simulink model "Day_09_Method1"  (R2024a)
settings: Solver=FixedStepAuto  StartTime=0.0  StopTime=10  FixedStep=0.01  RelTol=1e-3
values from neighbouring files (symbols this model uses):
  D0 = 2700    [Day_09.m]
  D1 = 2700    [Day_09.m]
  disturbance = 0    [Day_09.m]
  L0 = 0.01    [Day_09.m]
  L1 = 0.14    [Day_09.m]
  lim_theta = 2*pi    (= 6.28318530718)    [Day_09.m]
  lim_u = 1    [Day_09.m]
  lim_x = 1    [Day_09.m]
  M0 = L0*W0*T0*D0    (= 0.0027)    [Day_09.m]
  M1 = L1*W1*T1*D1    (= 0.0378)    [Day_09.m]
  M_c = 5    [Day_09.m]
  N_p = 50    [Day_09.m]
  num_state = 2    [Day_09.m]
  Q_Bar = kron(eye(N_p), Q)    [Day_09.m]
  R_Bar = kron(eye(M_c), R)    [Day_09.m]
  T0 = 0.01    [Day_09.m]
  T1 = 0.01    [Day_09.m]
  T_s = 0.01    [Day_09.m]
  Trajectory = zeros(num_state, 20000)    [Day_09.m]
  W0 = 0.01    [Day_09.m]
  W1 = 0.01    [Day_09.m]
undefined symbols (not defined in the file or in its folder): X, Y, Z
libraries: sm_lib x14, nesl_utility x7, simulink x1
settings Model: Creator=mingeun  LastModifiedBy=MinGeunPark
settings SolverCC: ZeroCrossAlgorithm=Adaptive
settings DataIOCC: ReturnWorkspaceOutputs=off
settings OptimizationCC: BlockReduction=off  DefaultParameterBehavior=Inlined  BufferReuse=off
settings DebuggingCC: IgnoredZcDiagnostic=none

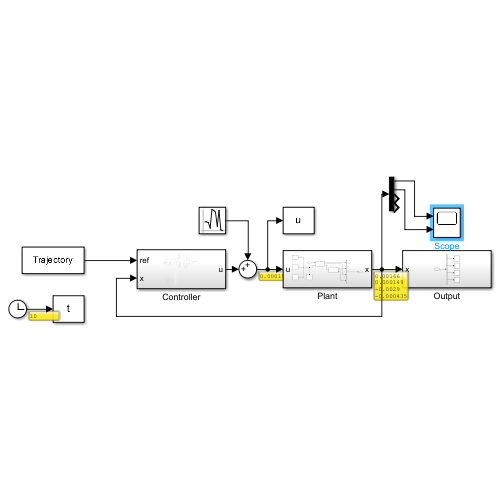
[thumbnail: Simulink's stored preview of the top-level diagram]
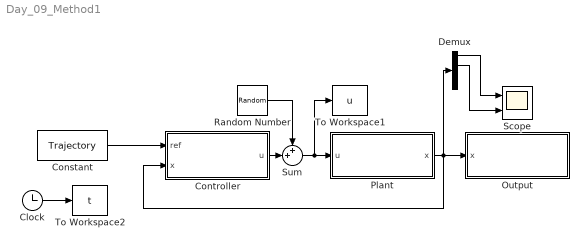
== system Day_09_Method1 ==
  Clock : Clock
  Constant : Constant  Value=Trajectory
  Controller : Subsystem
  Demux : Demux
  Output : Subsystem
  Plant : Subsystem
  Random Number : RandomNumber  Variance=0  SampleTime=T_s
  Scope : Scope  NumInputPorts=2
  Sum : Sum  Inputs=++|
  To Workspace1 : ToWorkspace  VariableName=u  SampleTime=-1
  To Workspace2 : ToWorkspace  VariableName=t  SampleTime=-1
  wires:
  Clock/1 -> To Workspace2/1
  Constant/1 -> Controller/1(ref)
  Plant/1(x) -> Demux/1, Controller/2(x), Output/1(x)
  Controller/1(u) -> Sum/2
  Sum/1 -> To Workspace1/1, Plant/1(u)
  Demux/1 -> Scope/1
  Demux/2 -> Scope/2
  Random Number/1 -> Sum/1

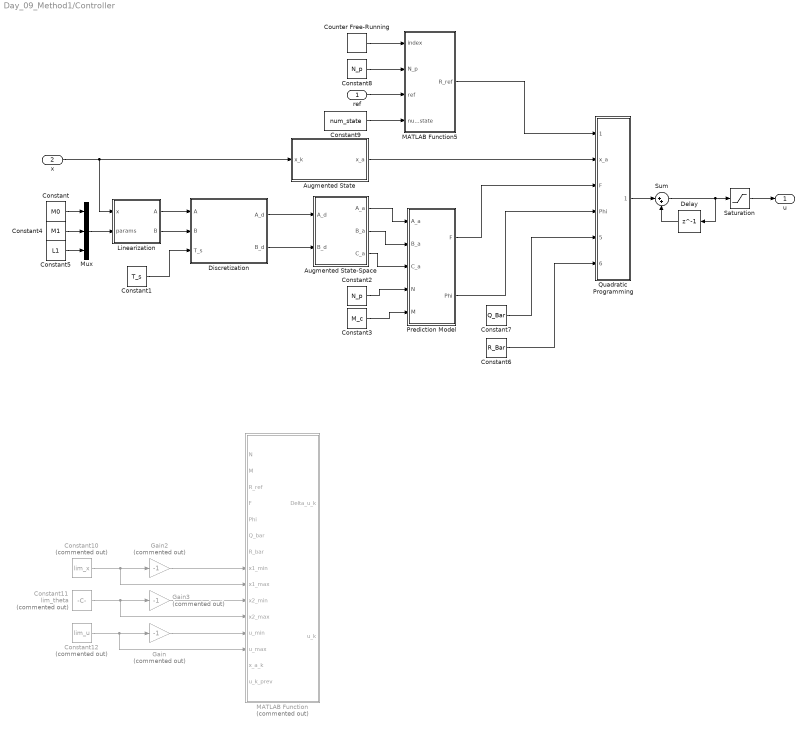
== system Day_09_Method1/Controller ==
  ref : Inport
  x : Inport  Port=2
  Augmented State : Subsystem
  Augmented State-Space : MATLAB Function  TreatAsAtomicUnit=on
  Constant : Constant  Value=M0
  Constant1 : Constant  Value=T_s
  Constant10 : Constant  Commented=on  Value=lim_x
  Constant11 : Constant  Commented=on  Value=lim_theta
  Constant12 : Constant  Commented=on  Value=lim_u
  Constant2 : Constant  Value=N_p
  Constant3 : Constant  Value=M_c
  Constant4 : Constant  Value=M1
  Constant5 : Constant  Value=L1
  Constant6 : Constant  Value=R_Bar
  Constant7 : Constant  Value=Q_Bar
  Constant8 : Constant  Value=N_p
  Constant9 : Constant  Value=num_state
  Counter Free-Running : simulink/Sources/Counter Free-Running  NumBits=32  tsamp=T_s
  Delay : Delay  DelayLength=1
  Discretization : Subsystem
  Gain : Gain  Commented=on  Gain=-1
  Gain2 : Gain  Commented=on  Gain=-1
  Gain3 : Gain  Commented=on  Gain=-1
  Linearization : MATLAB Function  TreatAsAtomicUnit=on
  MATLAB Function : MATLAB Function  Commented=on  TreatAsAtomicUnit=on
  MATLAB Function5 : MATLAB Function  TreatAsAtomicUnit=on
  Mux : Mux  Inputs=3
  Prediction Model : MATLAB Function  TreatAsAtomicUnit=on
  Quadratic Programming : Subsystem
  Saturation : Saturate  UpperLimit=lim_u  LowerLimit=-lim_u
  Sum : Sum  Inputs=|++
  u : Outport
  wires:
  Constant4/1 -> Mux/2
  Constant/1 -> Mux/1
  Sum/1 -> Saturation/1, Delay/1
  ref/1 -> MATLAB Function5/3(ref)
  Constant1/1 -> Discretization/3(T_s)
  Constant9/1 -> MATLAB Function5/4(num_state)
  Linearization/1(A) -> Discretization/1(A)
  Linearization/2(B) -> Discretization/2(B)
  Delay/1 -> Sum/2
  Prediction Model/2(Phi) -> Quadratic Programming/4(Phi)
  Augmented State/1(x_a) -> Quadratic Programming/2(x_a)
  Constant7/1 -> Quadratic Programming/5(Q_Bar)
  Counter Free-Running/1 -> MATLAB Function5/1(index)
  Constant8/1 -> MATLAB Function5/2(N_p)
  x/1 -> Linearization/1(x), Augmented State/1(x_k)
  MATLAB Function5/1(R_ref) -> Quadratic Programming/1(R_ref)
  Augmented State-Space/3(C_a) -> Prediction Model/3(C_a)
  Constant6/1 -> Quadratic Programming/6(R_Bar)
  Constant2/1 -> Prediction Model/4(N)
  Augmented State-Space/2(B_a) -> Prediction Model/2(B_a)
  Prediction Model/1(F) -> Quadratic Programming/3(F)
  Discretization/1(A_d) -> Augmented State-Space/1(A_d)
  Mux/1 -> Linearization/2(params)
  Augmented State-Space/1(A_a) -> Prediction Model/1(A_a)
  Discretization/2(B_d) -> Augmented State-Space/2(B_d)
  Constant3/1 -> Prediction Model/5(M)
  Constant5/1 -> Mux/3
  Constant12/1 -> MATLAB Function/13(u_max), Gain/1
  Constant10/1 -> MATLAB Function/9(x1_max), Gain2/1
  Gain2/1 -> MATLAB Function/8(x1_min)
  Gain3/1 -> MATLAB Function/10(x2_min)
  Constant11/1 -> MATLAB Function/11(x2_max), Gain3/1
  Gain/1 -> MATLAB Function/12(u_min)
  Saturation/1 -> u/1
  Quadratic Programming/1(Delta_u) -> Sum/1

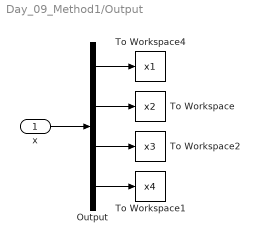
== system Day_09_Method1/Output ==
  x : Inport
  Output : Demux
  To Workspace : ToWorkspace  VariableName=x2  SampleTime=-1
  To Workspace1 : ToWorkspace  VariableName=x4  SampleTime=-1
  To Workspace2 : ToWorkspace  VariableName=x3  SampleTime=-1
  To Workspace4 : ToWorkspace  VariableName=x1  SampleTime=-1
  wires:
  Output/3 -> To Workspace2/1
  Output/4 -> To Workspace1/1
  Output/2 -> To Workspace/1
  Output/1 -> To Workspace4/1
  x/1 -> Output/1

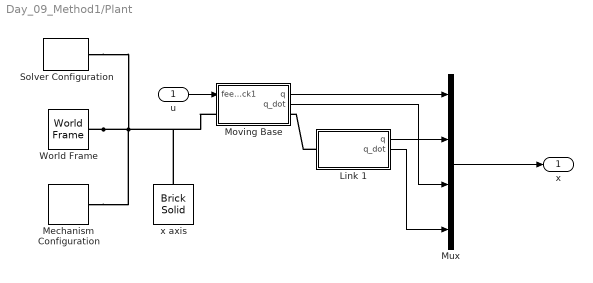
== system Day_09_Method1/Plant ==
  u : Inport
  Link 1 : Subsystem  mask{L=L1*100, W=W1*100, H=T1*100, rho=D1, rgb=[0.25 0.40 0.70], angle=0, F=disturbance}
      mask prompts: L "Length (cm)"; W "Width (cm)"; H "Thickness (cm)"; rho "Density (kg/m^3)"; rgb "Color [R G B]"; angle "Initial Angle (degree)"; F "Disturbance [N]"
  Mechanism Configuration : sm_lib/Utilities/Mechanism Configuration  UniformGravity=Constant  GravityVector=[0 0 -9.81]  GravityVectorUnits=m/s^2  LinearizationDelta=0.001  JointModeTransitionNonlinearIterations=2
  Moving Base : Subsystem  mask{L=L0*100, W=W0*100, H=T0*100, rho=D0, RGB=[0.8 0.45 0.0], x_init=0}
      mask prompts: L "Length (cm)"; W "Width (cm)"; H "Thickness (cm)"; rho "Density (kg/m^3)"; RGB "Color [R G B]"; x_init "x_init (cm)"
  Mux : Mux
  Solver Configuration : nesl_utility/Solver Configuration  PhysicalDomain=network_engine_domain  SubClassName=solver  LeftPortType=input  RightPortType=generic  Tones=[]  Harmonics=[]  SimulateNoise=off  Profile=off  UseLocalSampling=off  EnableSwitchedLinearOptims=on  FrequencyDomain=off  UseCCode=off  RelTol=0.001  AbsTol=0.001  MinStep=1e-09  ToWorkspace=off  RevertToSquareIcSolve=off  NumHomotopyIterations=100  PhasorMode=off  PhasorModeNumHarmonics=1  ConsistencySolver=NEWTON_XTOL_AFTER_FTOL  IndexReductionMethod=DerivativeReplacement  DoDC=off  ResidualTolerance=1e-09  ConsistencyTolSource=GLOBAL  ConsistencyAbsTol=0.001  ConsistencyRelTol=0.001  ConsistencyTolFactor=0.001  UseLocalSolver=off  LocalSolverChoice=NE_BACKWARD_EULER_ADVANCER  ResolveIndetEquations=on  FunctionEvalNumThread=1  LocalSolverSampleTime=0.001  DoFixedCost=off  MaxNonlinIter=3  MaxModeIter=2  ComputeImpulses=off  ImpulseIterations=2  LinearAlgebra=auto  LinearAlgebraNumThread=0  EquationFormulation=NE_TIME_EF  DelaysMemoryBudget=1024  AutomaticFiltering=on  FilteringTimeConstant=0.001  PartitionStorageMethod=AS_NEEDED  PartitionMemoryBudget=1024  PartitionMethod=ROBUST  MultibodyUseLocalSolver=off  MultibodyLocalSolverChoice=ODE1  MultibodyLocalSolverSampleTime=0.001
  World Frame : sm_lib/Frames and Transforms/World Frame
  x axis : sm_lib/Body Elements/Brick Solid  BrickDimensions=[1000 1 1]  BrickDimensionsUnits=mm  ExportEntireGeometry=off  InertiaType=CalculateFromGeometry  BasedOnType=Density  Density=1000  DensityUnits=kg/m^3  Mass=1  MassUnits=kg  CenterOfMass=[0 0 0]  CenterOfMassUnits=m  MomentsOfInertia=[1 1 1]  MomentsOfInertiaUnits=kg*m^2  ProductsOfInertia=[0 0 0]  ProductsOfInertiaUnits=kg*m^2  GraphicType=FromGeometry  MarkerShape=Sphere  MarkerSize=10  GraphicVisPropType=SimpleVisualProperties  GraphicDiffuseColor=[0.0 0.0 0.0]  GraphicOpacity=1  GraphicSpecularColor=[0.5 0.5 0.5 1.0]  GraphicAmbientColor=[0.15 0.15 0.15 1.0]  GraphicEmissiveColor=[0.0 0.0 0.0 1.0]  GraphicShininess=75  DoExposeReferenceFrame=on  SerializedFrames=<Frames/>
  x : Outport
  wires:
  Moving Base/1(q) -> Mux/1
  Link 1/1(q) -> Mux/2
  u/1 -> Moving Base/1(feedback1)
  Link 1/2(q_dot) -> Mux/4
  Moving Base/2(q_dot) -> Mux/3
  Mux/1 -> x/1
  connections:
  World Frame/RConn1 -- Solver Configuration/RConn1 -- Moving Base/LConn1 -- x axis/RConn1 -- Mechanism Configuration/RConn1
  Link 1/LConn1 -- Moving Base/RConn1

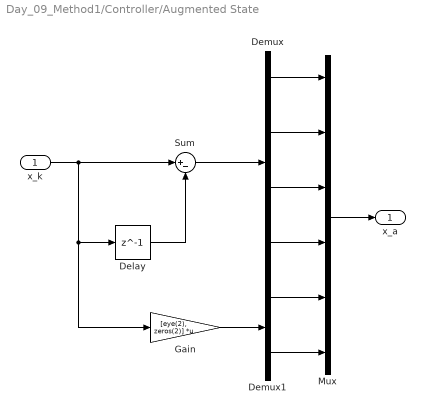
== system Day_09_Method1/Controller/Augmented State ==
  x_k : Inport
  Delay : Delay  DelayLength=1
  Demux : Demux
  Demux1 : Demux  Outputs=2
  Gain : Gain  Gain=[eye(2), zeros(2)]  Multiplication=Matrix(K*u) (u vector)
  Mux : Mux  Inputs=6
  Sum : Sum  Inputs=|+-
  x_a : Outport
  wires:
  x_k/1 -> Sum/1, Gain/1, Delay/1
  Sum/1 -> Demux/1
  Demux/1 -> Mux/1
  Demux/2 -> Mux/2
  Demux/3 -> Mux/3
  Demux/4 -> Mux/4
  Demux1/1 -> Mux/5
  Demux1/2 -> Mux/6
  Mux/1 -> x_a/1
  Delay/1 -> Sum/2
  Gain/1 -> Demux1/1

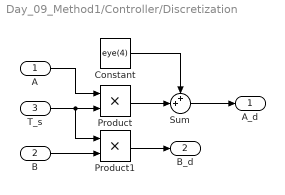
== system Day_09_Method1/Controller/Discretization ==
  A : Inport
  B : Inport  Port=2
  T_s : Inport  Port=3
  Constant : Constant  Value=eye(4)
  Product : Product
  Product1 : Product
  Sum : Sum  Inputs=++|
  A_d : Outport
  B_d : Outport  Port=2
  wires:
  Sum/1 -> A_d/1
  Product1/1 -> B_d/1
  Constant/1 -> Sum/1
  B/1 -> Product1/2
  T_s/1 -> Product1/1, Product/2
  Product/1 -> Sum/2
  A/1 -> Product/1

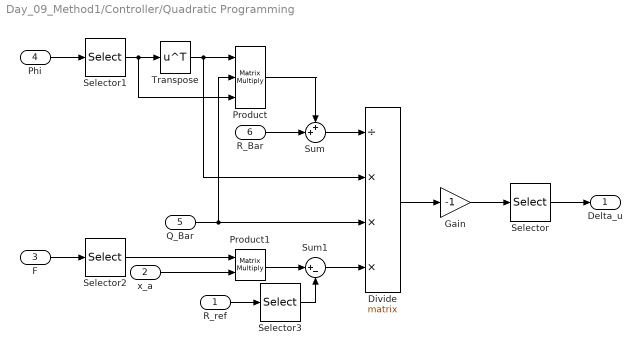
== system Day_09_Method1/Controller/Quadratic Programming ==
  R_ref : Inport
  x_a : Inport  Port=2
  F : Inport  Port=3
  Phi : Inport  Port=4
  Q_Bar : Inport  Port=5
  R_Bar : Inport  Port=6
  Divide : Product  Inputs=/***  Multiplication=Matrix(*)
  Gain : Gain  Gain=-1
  Product : Product  Inputs=3  Multiplication=Matrix(*)
  Product1 : Product  Multiplication=Matrix(*)
  Selector : Selector  InputPortWidth=M_c  IndexOptions=Index vector (dialog)  Indices=1  OutputSizes=1
  Selector1 : Selector  NumberOfDimensions=2  InputPortWidth=3  IndexOptions=Index vector (dialog),Index vector (dialog)  Indices=[1:N_p*num_state],[1:M_c]  OutputSizes=1,1
  Selector2 : Selector  NumberOfDimensions=2  InputPortWidth=3  IndexOptions=Index vector (dialog),Index vector (dialog)  Indices=[1:N_p*num_state],[1:4 + num_state]  OutputSizes=1,1
  Selector3 : Selector  NumberOfDimensions=2  InputPortWidth=N_p*2  IndexOptions=Index vector (dialog),Index vector (dialog)  Indices=[1:N_p*num_state],1  OutputSizes=1,1
  Sum : Sum  Inputs=++|
  Sum1 : Sum  Inputs=|+-
  Transpose : Math  Operator=transpose
  Delta_u : Outport
  wires:
  Selector/1 -> Delta_u/1
  Gain/1 -> Selector/1
  Divide/1 -> Gain/1
  Sum1/1 -> Divide/4
  Product1/1 -> Sum1/1
  Sum/1 -> Divide/1
  R_Bar/1 -> Sum/2
  F/1 -> Selector2/1
  Product/1 -> Sum/1
  Q_Bar/1 -> Product/2, Divide/3
  Transpose/1 -> Divide/2, Product/1
  Phi/1 -> Selector1/1
  Selector1/1 -> Product/3, Transpose/1
  Selector2/1 -> Product1/1
  R_ref/1 -> Selector3/1
  Selector3/1 -> Sum1/2
  x_a/1 -> Product1/2

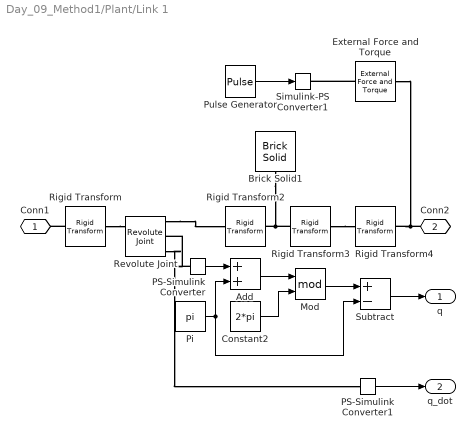
== system Day_09_Method1/Plant/Link 1 ==
  Add : Sum
  Brick Solid1 : sm_lib/Body Elements/Brick Solid  BrickDimensions=[L W H]  BrickDimensionsUnits=cm  ExportEntireGeometry=off  InertiaType=CalculateFromGeometry  BasedOnType=Density  Density=rho  DensityUnits=kg/m^3  Mass=1  MassUnits=kg  CenterOfMass=[0 0 0]  CenterOfMassUnits=m  MomentsOfInertia=[1 1 1]  MomentsOfInertiaUnits=kg*m^2  ProductsOfInertia=[0 0 0]  ProductsOfInertiaUnits=kg*m^2  GraphicType=FromGeometry  MarkerShape=Sphere  MarkerSize=10  GraphicVisPropType=SimpleVisualProperties  GraphicDiffuseColor=rgb  GraphicOpacity=1  GraphicSpecularColor=[0.5 0.5 0.5 1.0]  GraphicAmbientColor=[0.15 0.15 0.15 1.0]  GraphicEmissiveColor=[0.0 0.0 0.0 1.0]  GraphicShininess=75  DoExposeReferenceFrame=on  SerializedFrames=<Frames/>
  Constant2 : Constant  Value=2*pi
  External Force and Torque : sm_lib/Forces and Torques/External Force and Torque  EnableForceX=on  EnableForceY=off  EnableForceZ=off  EnableForce=off  ForceResolutionFrame=World  EnableTorqueX=off  EnableTorqueY=off  EnableTorqueZ=off  EnableTorque=off  TorqueResolutionFrame=World
  Mod : Math  Operator=mod  OutputSignalType=real
  PS-Simulink Converter : nesl_utility/PS-Simulink Converter  PhysicalDomain=network_engine_domain  SubClassName=ps_output  LeftPortType=input  RightPortType=output  PseudoPeriodic=off  Frequencies=[]  VectorFormat=inherit  Unit=inherit  AffineConversion=off
  PS-Simulink Converter1 : nesl_utility/PS-Simulink Converter  PhysicalDomain=network_engine_domain  SubClassName=ps_output  LeftPortType=input  RightPortType=output  PseudoPeriodic=off  Frequencies=[]  VectorFormat=inherit  Unit=inherit  AffineConversion=off
  Pi : Constant  Value=pi  OutDataTypeStr=Inherit: Inherit via back propagation
  Pulse Generator : DiscretePulseGenerator  PulseType=Time based  Amplitude=F  Period=1000000  PulseWidth=1/1000000  PhaseDelay=0.25
  Revolute Joint : sm_lib/Joints/Revolute Joint  JointMode=Normal  CompositeWrenchDir=FollowerOnBase  CompositeWrenchFrame=BaseFrame  SenseConstraintForce=off  SenseConstraintTorque=off  SenseTotalForce=off  SenseTotalTorque=off  PositionTargetSpecify=on  PositionTargetPriority=High  PositionTargetValue=angle  PositionTargetValueUnits=deg  VelocityTargetSpecify=off  VelocityTargetPriority=High  VelocityTargetValue=0  VelocityTargetValueUnits=deg/s  EquilibriumPosition=0  EquilibriumPositionUnits=deg  SpringStiffness=0  SpringStiffnessUnits=N*m/deg  DampingCoefficient=0  DampingCoefficientUnits=N*m/(deg/s)  LowerLimitSpecify=off  LowerLimitBound=-90  LowerLimitBoundUnits=deg  LowerLimitStiffness=1e4  LowerLimitStiffnessUnits=N*m/deg  LowerLimitDamping=10  LowerLimitDampingUnits=N*m/(deg/s)  LowerLimitTransitionRegionWidth=0.1  LowerLimitTransitionRegionWidthUnits=deg  UpperLimitSpecify=off  UpperLimitBound=90  UpperLimitBoundUnits=deg  UpperLimitStiffness=1e4  UpperLimitStiffnessUnits=N*m/deg  UpperLimitDamping=10  UpperLimitDampingUnits=N*m/(deg/s)  UpperLimitTransitionRegionWidth=0.1  UpperLimitTransitionRegionWidthUnits=deg  TorqueActuationMode=InputTorque  MotionActuationMode=ComputedMotion  SensePosition=on  SenseVelocity=on  SenseAcceleration=off  SenseTorqueForce=off  SenseLowerLimitTorqueForce=off  SenseUpperLimitTorqueForce=off
  Rigid Transform : sm_lib/Frames and Transforms/Rigid Transform  RotationMethod=RotationMatrix  FollAlignAxisA=+X  BaseAlignAxisA=+Y  FollAlignAxisB=+Y  BaseAlignAxisB=+Z  RotationStandardAxis=+X  RotationAngle=90  RotationAngleUnits=deg  RotationArbitraryAxis=[0 0 1]  RotationSequenceAxes=FollowerAxes  RotationSequence=XYX  RotationSequenceAngles=[0 0 0]  RotationSequenceAnglesUnits=deg  RotationMatrix=[0 0 1; -1 0 0; 0 -1 0]  Quaternion=[1 0 0 0]  TranslationMethod=None  TranslationCartesianOffset=[0 0 0]  TranslationCartesianOffsetUnits=m  TranslationStandardAxis=+Z  TranslationStandardOffset=0  TranslationStandardOffsetUnits=m  TranslationROffset=0  TranslationROffsetUnits=m  TranslationThetaOffset=0  TranslationThetaOffsetUnits=deg  TranslationZOffset=0  TranslationZOffsetUnits=m
  Rigid Transform2 : sm_lib/Frames and Transforms/Rigid Transform  RotationMethod=None  FollAlignAxisA=+X  BaseAlignAxisA=+Y  FollAlignAxisB=+Y  BaseAlignAxisB=+Z  RotationStandardAxis=+Z  RotationAngle=0  RotationAngleUnits=deg  RotationArbitraryAxis=[0 0 1]  RotationSequenceAxes=FollowerAxes  RotationSequence=XYX  RotationSequenceAngles=[0 0 0]  RotationSequenceAnglesUnits=deg  RotationMatrix=[1 0 0;0 1 0;0 0 1]  Quaternion=[1 0 0 0]  TranslationMethod=StandardAxis  TranslationCartesianOffset=[0 0 0]  TranslationCartesianOffsetUnits=m  TranslationStandardAxis=-X  TranslationStandardOffset=L/2  TranslationStandardOffsetUnits=cm  TranslationROffset=0  TranslationROffsetUnits=m  TranslationThetaOffset=0  TranslationThetaOffsetUnits=deg  TranslationZOffset=0  TranslationZOffsetUnits=m
  Rigid Transform3 : sm_lib/Frames and Transforms/Rigid Transform  RotationMethod=None  FollAlignAxisA=+X  BaseAlignAxisA=+Y  FollAlignAxisB=+Y  BaseAlignAxisB=+Z  RotationStandardAxis=+Z  RotationAngle=0  RotationAngleUnits=deg  RotationArbitraryAxis=[0 0 1]  RotationSequenceAxes=FollowerAxes  RotationSequence=XYX  RotationSequenceAngles=[0 0 0]  RotationSequenceAnglesUnits=deg  RotationMatrix=[1 0 0;0 1 0;0 0 1]  Quaternion=[1 0 0 0]  TranslationMethod=StandardAxis  TranslationCartesianOffset=[0 0 0]  TranslationCartesianOffsetUnits=m  TranslationStandardAxis=-X  TranslationStandardOffset=L/2  TranslationStandardOffsetUnits=cm  TranslationROffset=0  TranslationROffsetUnits=m  TranslationThetaOffset=0  TranslationThetaOffsetUnits=deg  TranslationZOffset=0  TranslationZOffsetUnits=m
  Rigid Transform4 : sm_lib/Frames and Transforms/Rigid Transform  RotationMethod=None  FollAlignAxisA=+X  BaseAlignAxisA=+Y  FollAlignAxisB=+Y  BaseAlignAxisB=+Z  RotationStandardAxis=+Z  RotationAngle=0  RotationAngleUnits=deg  RotationArbitraryAxis=[0 0 1]  RotationSequenceAxes=FollowerAxes  RotationSequence=XYX  RotationSequenceAngles=[0 0 0]  RotationSequenceAnglesUnits=deg  RotationMatrix=[1 0 0; 0 0 1; 0 -1 0]  Quaternion=[1 0 0 0]  TranslationMethod=StandardAxis  TranslationCartesianOffset=[0 0 0]  TranslationCartesianOffsetUnits=m  TranslationStandardAxis=+X  TranslationStandardOffset=L  TranslationStandardOffsetUnits=cm  TranslationROffset=0  TranslationROffsetUnits=m  TranslationThetaOffset=0  TranslationThetaOffsetUnits=deg  TranslationZOffset=0  TranslationZOffsetUnits=m
  Simulink-PS Converter1 : nesl_utility/Simulink-PS Converter  PhysicalDomain=network_engine_domain  SubClassName=ps_input  LeftPortType=input  RightPortType=output  PseudoPeriodic=off  Frequencies=[]  NoiseDistribution=none  NoiseParameters=[]  Unit=1  AffineConversion=off  FilteringAndDerivatives=provide  SimscapeFilterOrder=1  InputFilterTimeConstant=0.001  UdotUserProvided=0
  Subtract : Sum  Inputs=+-
  Conn1 : PMIOPort  Side=Left
  Conn2 : PMIOPort  Port=2  Side=Right
  q : Outport
  q_dot : Outport  Port=2
  wires:
  Pulse Generator/1 -> Simulink-PS Converter1/1
  Mod/1 -> Subtract/1
  Constant2/1 -> Mod/2
  Pi/1 -> Subtract/2, Add/2
  PS-Simulink Converter/1 -> Add/1
  Add/1 -> Mod/1
  Subtract/1 -> q/1
  PS-Simulink Converter1/1 -> q_dot/1
  connections:
  PS-Simulink Converter/LConn1 -- Revolute Joint/RConn2
  Rigid Transform3/RConn1 -- Rigid Transform4/LConn1
  Rigid Transform/LConn1 -- Revolute Joint/LConn1
  Rigid Transform3/LConn1 -- Brick Solid1/RConn1 -- Rigid Transform2/LConn1
  Conn2/RConn1 -- External Force and Torque/RConn1 -- Rigid Transform4/RConn1
  Rigid Transform/RConn1 -- Conn1/RConn1
  Revolute Joint/RConn1 -- Rigid Transform2/RConn1
  External Force and Torque/LConn1 -- Simulink-PS Converter1/RConn1
  Revolute Joint/RConn3 -- PS-Simulink Converter1/LConn1

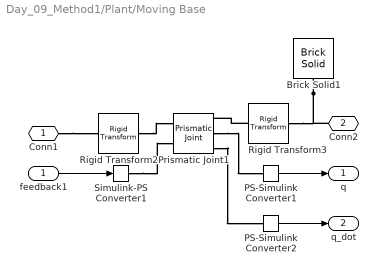
== system Day_09_Method1/Plant/Moving Base ==
  feedback1 : Inport
  Brick Solid1 : sm_lib/Body Elements/Brick Solid  BrickDimensions=[L W H]  BrickDimensionsUnits=cm  ExportEntireGeometry=off  InertiaType=CalculateFromGeometry  BasedOnType=Density  Density=rho  DensityUnits=kg/m^3  Mass=1  MassUnits=kg  CenterOfMass=[0 0 0]  CenterOfMassUnits=m  MomentsOfInertia=[1 1 1]  MomentsOfInertiaUnits=kg*m^2  ProductsOfInertia=[0 0 0]  ProductsOfInertiaUnits=kg*m^2  GraphicType=FromGeometry  MarkerShape=Sphere  MarkerSize=10  GraphicVisPropType=SimpleVisualProperties  GraphicDiffuseColor=RGB  GraphicOpacity=1  GraphicSpecularColor=[0.5 0.5 0.5 1.0]  GraphicAmbientColor=[0.15 0.15 0.15 1.0]  GraphicEmissiveColor=[0.0 0.0 0.0 1.0]  GraphicShininess=75  DoExposeReferenceFrame=on  SerializedFrames=<Frames/>
  PS-Simulink Converter1 : nesl_utility/PS-Simulink Converter  PhysicalDomain=network_engine_domain  SubClassName=ps_output  LeftPortType=input  RightPortType=output  PseudoPeriodic=off  Frequencies=[]  VectorFormat=inherit  Unit=inherit  AffineConversion=off
  PS-Simulink Converter2 : nesl_utility/PS-Simulink Converter  PhysicalDomain=network_engine_domain  SubClassName=ps_output  LeftPortType=input  RightPortType=output  PseudoPeriodic=off  Frequencies=[]  VectorFormat=inherit  Unit=inherit  AffineConversion=off
  Prismatic Joint1 : sm_lib/Joints/Prismatic Joint  JointMode=Normal  CompositeWrenchDir=FollowerOnBase  CompositeWrenchFrame=BaseFrame  SenseConstraintForce=off  SenseConstraintTorque=off  SenseTotalForce=off  SenseTotalTorque=off  PositionTargetSpecify=on  PositionTargetPriority=High  PositionTargetValue=x_init  PositionTargetValueUnits=cm  VelocityTargetSpecify=off  VelocityTargetPriority=High  VelocityTargetValue=0  VelocityTargetValueUnits=m/s  EquilibriumPosition=0  EquilibriumPositionUnits=m  SpringStiffness=0  SpringStiffnessUnits=N/m  DampingCoefficient=0  DampingCoefficientUnits=N/(m/s)  LowerLimitSpecify=off  LowerLimitBound=-.5  LowerLimitBoundUnits=m  LowerLimitStiffness=1e6  LowerLimitStiffnessUnits=N/m  LowerLimitDamping=1e3  LowerLimitDampingUnits=N/(m/s)  LowerLimitTransitionRegionWidth=1e-4  LowerLimitTransitionRegionWidthUnits=m  UpperLimitSpecify=off  UpperLimitBound=.5  UpperLimitBoundUnits=m  UpperLimitStiffness=1e6  UpperLimitStiffnessUnits=N/m  UpperLimitDamping=1e3  UpperLimitDampingUnits=N/(m/s)  UpperLimitTransitionRegionWidth=1e-4  UpperLimitTransitionRegionWidthUnits=m  TorqueActuationMode=InputTorque  MotionActuationMode=ComputedMotion  SensePosition=on  SenseVelocity=on  SenseAcceleration=off  SenseTorqueForce=off  SenseLowerLimitTorqueForce=off  SenseUpperLimitTorqueForce=off
  Rigid Transform2 : sm_lib/Frames and Transforms/Rigid Transform  RotationMethod=StandardAxis  FollAlignAxisA=+X  BaseAlignAxisA=+Y  FollAlignAxisB=+Y  BaseAlignAxisB=+Z  RotationStandardAxis=+Y  RotationAngle=90  RotationAngleUnits=deg  RotationArbitraryAxis=[0 0 1]  RotationSequenceAxes=FollowerAxes  RotationSequence=XYX  RotationSequenceAngles=[0 0 0]  RotationSequenceAnglesUnits=deg  RotationMatrix=[1 0 0;0 1 0;0 0 1]  Quaternion=[1 0 0 0]  TranslationMethod=None  TranslationCartesianOffset=[0 0 0]  TranslationCartesianOffsetUnits=m  TranslationStandardAxis=+Z  TranslationStandardOffset=0  TranslationStandardOffsetUnits=m  TranslationROffset=0  TranslationROffsetUnits=m  TranslationThetaOffset=0  TranslationThetaOffsetUnits=deg  TranslationZOffset=0  TranslationZOffsetUnits=m
  Rigid Transform3 : sm_lib/Frames and Transforms/Rigid Transform  RotationMethod=StandardAxis  FollAlignAxisA=+X  BaseAlignAxisA=+Y  FollAlignAxisB=+Y  BaseAlignAxisB=+Z  RotationStandardAxis=+Y  RotationAngle=90  RotationAngleUnits=deg  RotationArbitraryAxis=[0 0 1]  RotationSequenceAxes=FollowerAxes  RotationSequence=XYX  RotationSequenceAngles=[0 0 0]  RotationSequenceAnglesUnits=deg  RotationMatrix=[1 0 0;0 1 0;0 0 1]  Quaternion=[1 0 0 0]  TranslationMethod=None  TranslationCartesianOffset=[0 0 0]  TranslationCartesianOffsetUnits=m  TranslationStandardAxis=+Z  TranslationStandardOffset=0  TranslationStandardOffsetUnits=m  TranslationROffset=0  TranslationROffsetUnits=m  TranslationThetaOffset=0  TranslationThetaOffsetUnits=deg  TranslationZOffset=0  TranslationZOffsetUnits=m
  Simulink-PS Converter1 : nesl_utility/Simulink-PS Converter  PhysicalDomain=network_engine_domain  SubClassName=ps_input  LeftPortType=input  RightPortType=output  PseudoPeriodic=off  Frequencies=[]  NoiseDistribution=none  NoiseParameters=[]  Unit=1  AffineConversion=off  FilteringAndDerivatives=provide  SimscapeFilterOrder=1  InputFilterTimeConstant=0.001  UdotUserProvided=0
  Conn1 : PMIOPort  Side=Left
  Conn2 : PMIOPort  Port=2  Side=Right
  q : Outport
  q_dot : Outport  Port=2
  wires:
  feedback1/1 -> Simulink-PS Converter1/1
  PS-Simulink Converter1/1 -> q/1
  PS-Simulink Converter2/1 -> q_dot/1
  connections:
  Brick Solid1/RConn1 -- Conn2/RConn1 -- Rigid Transform3/LConn1
  Rigid Transform2/RConn1 -- Prismatic Joint1/LConn1
  Prismatic Joint1/RConn2 -- PS-Simulink Converter1/LConn1
  Simulink-PS Converter1/RConn1 -- Prismatic Joint1/LConn2
  Conn1/RConn1 -- Rigid Transform2/LConn1
  Rigid Transform3/RConn1 -- Prismatic Joint1/RConn1
  Prismatic Joint1/RConn3 -- PS-Simulink Converter2/LConn1

== matlab function Day_09_Method1/Controller/MATLAB Function ==
  data: Delta_u_k output; N input; M input; R_ref input; F input; Phi input; Q_bar input; R_bar input; x1_min input; x1_max input; x2_min input; x2_max input; u_min input; u_max input; x_a_k input; u_k_prev input; u_k output
function [Delta_u_k, u_k] = optimal_control(N, M, R_ref, F, Phi, Q_bar, R_bar, x1_min, x1_max, x2_min, x2_max, u_min, u_max, x_a_k, u_k_prev)
    % Define the number of states and inputs
    n_x = 6;
    n_u = 1;

    R_ref = R_ref(1:N*2);
    Phi = Phi(1:N*2, 1:M);
    F = F(1:N*2, 1:6);

    % Calculate the Hessian matrix H and the linear term f
    Phi_t_Q_Phi = Phi' * Q_bar * Phi;
    H = 2 * (Phi_t_Q_Phi + R_bar);  % The Hessian matrix

    f = 2 * Phi' * Q_bar * (F * x_a_k - R_ref);  % Linear term
    
    % Separate odd and even rows for expected output
    expected_output_x1 = F(1:2:end, :) * x_a_k;  % Odd rows (corresponding to x1)
    expected_output_x2 = F(2:2:end, :) * x_a_k;  % Even rows (corresponding to x2)
    
    % Separate Phi into odd and even rows
    Phi_x1 = Phi(1:2:end, :);  % Odd rows for x1
    Phi_x2 = Phi(2:2:end, :);  % Even rows for x2
    
    % Formulate the input constraints
    A_ineq_input = [eye(M * n_u); -eye(M * n_u)];
    b_ineq_input = [repmat(u_max, M * n_u, 1); repmat(-u_min, M * n_u, 1)];
    
    % Formulate the output constraints for x1 and x2 separately
    A_ineq_output_x1 = [Phi_x1; -Phi_x1];
    b_ineq_output_x1 = [repmat(x1_max, N, 1) - expected_output_x1;
                        repmat(-x1_min, N, 1) + expected_output_x1];
    
    A_ineq_output_x2 = [Phi_x2; -Phi_x2];
    b_ineq_output_x2 = [repmat(x2_max, N, 1) - expected_output_x2;
                        repmat(-x2_min, N, 1) + expected_output_x2];
    
    % Combine all constraints
    A_ineq = [A_ineq_input; A_ineq_output_x1; A_ineq_output_x2];
    b_ineq = [b_ineq_input; b_ineq_output_x1; b_ineq_output_x2];

    % Initial guess for Delta_U (can be zeros or based on the previous solution)
    Delta_U0 = zeros(M * n_u, 1);  % Start with zeros

    % Solve the QP problem using quadprog
    options = optimoptions('quadprog', 'Algorithm', 'active-set', 'Display', 'off');
    [Delta_U, ~, exitflag] = quadprog(H, f, A_ineq, b_ineq, [], [], [], [], Delta_U0, options);

    if exitflag == 1
        Delta_u_k = Delta_U(1:n_u);  % The first control input increment
        u_k = u_k_prev + Delta_u_k;  % Calculate the actual control input
    else
        error('quadprog did not converge');
    end
end

== matlab function Day_09_Method1/Controller/Linearization ==
  data: x input; A output; params input; B output
function [A, B] = fcn(x, params)
x1 = x(1);
x2 = x(2);
x3 = x(3);
x4 = x(4);

m0 = params(1);
m1 = params(2);
l1 = params(3);

g = 9.81;

A = [0, 0, 1, 0;
     0, 0, 0, 1;
     0, (m1*cos(x2)*(3*g*cos(x2) - 2*l1*x4^2))/(4*m0 + 4*m1 - 3*m1*cos(x2)^2) - (3*g*m1*sin(x2)^2)/(4*m0 + 4*m1 - 3*m1*cos(x2)^2) - (6*m1^2*cos(x2)*sin(x2)^2*(3*g*cos(x2) - 2*l1*x4^2))/(4*m0 + 4*m1 - 3*m1*cos(x2)^2)^2, 0, -(4*l1*m1*sin(x2)*x4)/(4*m0 + 4*m1 - 3*m1*cos(x2)^2);
     0, (3*m1*sin(x2)^2*x4^2)/(4*m0 + 4*m1 - 3*m1*cos(x2)^2) + (3*cos(x2)*(2*g*m0 + 2*g*m1 - l1*m1*cos(x2)*x4^2))/(l1*(4*m0 + 4*m1 - 3*m1*cos(x2)^2)) - (18*m1*cos(x2)*sin(x2)^2*(2*g*m0 + 2*g*m1 - l1*m1*cos(x2)*x4^2))/(l1*(4*m0 + 4*m1 - 3*m1*cos(x2)^2)^2), 0, -(6*m1*cos(x2)*sin(x2)*x4)/(4*m0 + 4*m1 - 3*m1*cos(x2)^2)];

B = [0;
     0;
     4/(4*m0 + 4*m1 - 3*m1*cos(x2)^2);
     (6*cos(x2))/(4*l1*m0 + 4*l1*m1 - 3*l1*m1*cos(x2)^2)];

== matlab function Day_09_Method1/Controller/Augmented State-Space ==
  data: A_d input; A_a output; B_d input; B_a output; C_a output
function [A_a, B_a, C_a] = fcn(A_d, B_d)

C_d = eye(2, 4);

[m, n] = size(C_d);
[~, o] = size(B_d);

A_a = eye(m+n, m+n);
A_a(1:n ,1:n) = A_d;
A_a(n+1:n+m, 1:n) = C_d*A_d;

B_a = zeros(n+m, o);
B_a(1:n, :) = B_d;
B_a(n+1:n+m, :) = C_d*B_d;

C_a = zeros(m, n+m);
C_a(:, n+1:n+m) = eye(m, m);

== matlab function Day_09_Method1/Controller/Prediction Model ==
  data: A_a input; F output [1..100]; B_a input; C_a input; N input; M input; Phi output [1..100]
function [F, Phi] = fcn(A_a, B_a, C_a, N, M)

[m_A, n_A] = size(A_a);
[m_C, n_C] = size(C_a);

% F = zeros(N*m_C, n_A);
% h = zeros(N*m_C, n_A);

F = zeros(1000, 6);
h = zeros(1000, 6);

F(1:2, :) = C_a*A_a;
h(1:2, :) = C_a;

for i = 2 : N
    F(i*2-1:i*2, :) = F((i-1)*2-1:(i-1)*2,:)*A_a;
    h(i*2-1:i*2, :) = h((i-1)*2-1:(i-1)*2,:)*A_a;
end

v = h * B_a;
% Phi = zeros(N*2, M);
Phi = zeros(1000, 50);
Phi(:, 1) = v;

for i = 2 : M
    Phi(1:N*2, i) = [zeros(2*(i-1), 1); v(1:2*(N-i+1), 1)];
end

== matlab function Day_09_Method1/Controller/MATLAB Function5 ==
  data: index input; N_p input; ref input; R_ref output [1..100]; num_state input
function R_ref = sliding_window(index, N_p, ref, num_state)
    index = index + 1;
    % x = zeros(2, N_p);
    x = zeros(num_state, 1000/num_state);
    x(:, 1:N_p) = ref(:, index:index+N_p-1);
    R_ref = reshape(x, 1000, 1);
end
